simulink model "p1"  (R2024a)
settings: Solver=VariableStepAuto  StartTime=0.0  StopTime=10.0  RelTol=1e-3
settings Model: Creator=majidsadeghinejad  LastModifiedBy=majidsadeghinejad

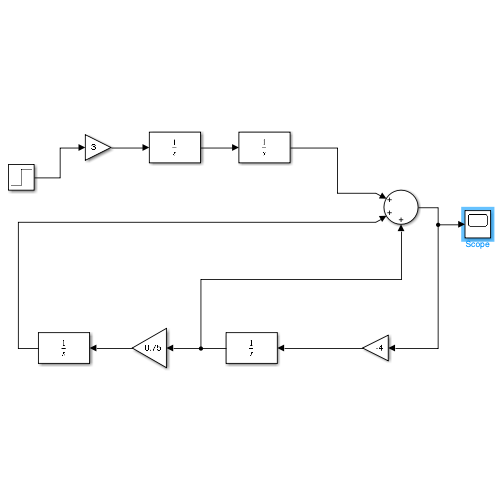
[thumbnail: Simulink's stored preview of the top-level diagram]
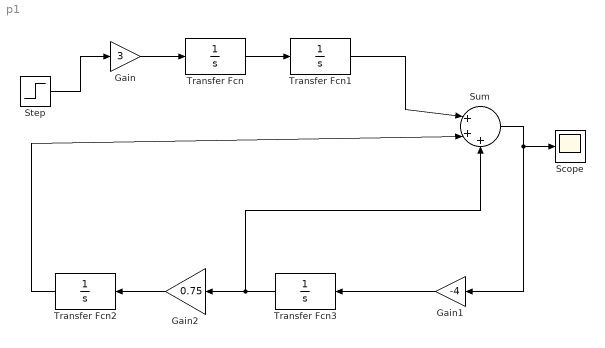
== system p1 ==
  Gain : Gain  Gain=3
  Gain1 : Gain  Gain=-4
  Gain2 : Gain  Gain=0.75
  Scope : Scope
  Step : Step  Time=0  SampleTime=0
  Sum : Sum  Inputs=|+++
  Transfer Fcn{,1..3} (4 alike) : TransferFcn  Denominator=[1 0]
  wires:
  Transfer Fcn/1 -> Transfer Fcn1/1
  Gain/1 -> Transfer Fcn/1
  Transfer Fcn1/1 -> Sum/1
  Sum/1 -> Gain1/1, Scope/1
  Gain2/1 -> Transfer Fcn2/1
  Transfer Fcn3/1 -> Sum/3, Gain2/1
  Gain1/1 -> Transfer Fcn3/1
  Transfer Fcn2/1 -> Sum/2
  Step/1 -> Gain/1
